simulink model "state_fb_xfer"  (Simulink 8.6)
settings: Solver=ode45  StartTime=0.0  StopTime=5  MaxStep=0.001  RelTol=1e-3
settings Model: Creator=Thomas Chmielewski  LastModifiedBy=DR_C
settings OptimizationCC: InitFltsAndDblsToZero=on
settings DebuggingCC: SaveWithParameterizedLinksMsg=none  SignalResolutionControl=TryResolveAllWithWarning  SolverPrmCheckMsg=none  MultiTaskDSMMsg=warning  MultiTaskCondExecSysMsg=none  FcnCallInpInsideContextMsg=UseLocalSettings  StrictBusMsg=None
settings HardwareCC: TargetUnknown=on
settings GRTTargetCC: TargetFcnLib=ansi_tfl_tmw.mat  GeneratePreprocessorConditionals=Use local settings

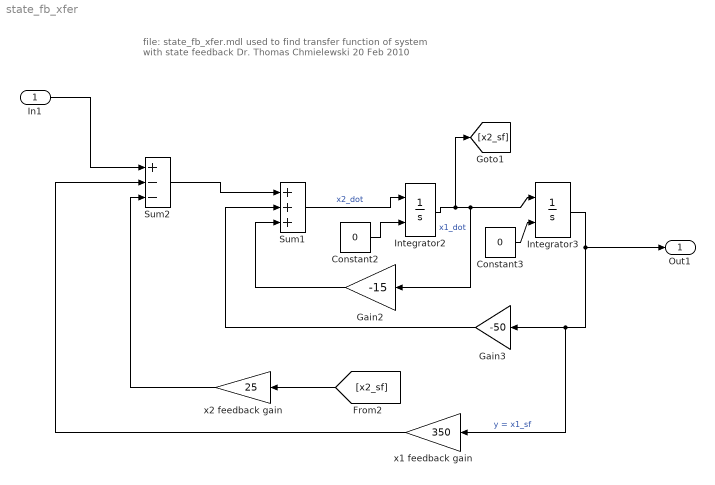
== system state_fb_xfer ==
  note: file:  state_fb_xfer.mdl
      | used to find transfer function of system with state feedback
      |
      | Dr. Thomas Chmielewski
      | 20 Feb 2010
  In1 : Inport
  Constant2 : Constant  Value=0
  Constant3 : Constant  Value=0
  Gain2 : Gain  Gain=-15
  Gain3 : Gain  Gain=-50
  Integrator2 : Integrator  InitialConditionSource=external  InitialCondition=1
  Integrator3 : Integrator  InitialConditionSource=external  InitialCondition=10
  Sum1 : Sum  Inputs=+++
  Sum2 : Sum  Inputs=+--
  x1 feedback gain : Gain  Gain=350
  x2 feedback gain : Gain  Gain=25
  Out1 : Outport
  wires:
  Integrator2/1 -> Integrator3/1, Gain2/1, [x2_sf]  "x1_dot"
  Sum1/1 -> Integrator2/1  "x2_dot"
  Integrator3/1 -> Gain3/1, x1 feedback gain/1, Out1/1  "y = x1_sf"
  Gain2/1 -> Sum1/3
  Gain3/1 -> Sum1/2
  Constant2/1 -> Integrator2/2
  Constant3/1 -> Integrator3/2
  Sum2/1 -> Sum1/1
  x2 feedback gain/1 -> Sum2/3
  x1 feedback gain/1 -> Sum2/2
  [x2_sf] -> x2 feedback gain/1
  In1/1 -> Sum2/1
